simulink model "Problem_8"  (R2020b)
settings: Solver=VariableStepAuto  StartTime=0.0  StopTime=inf  RelTol=1e-3
settings Model: PacingRate=0.028000  Creator=vigne  LastModifiedBy=Yeshwanth

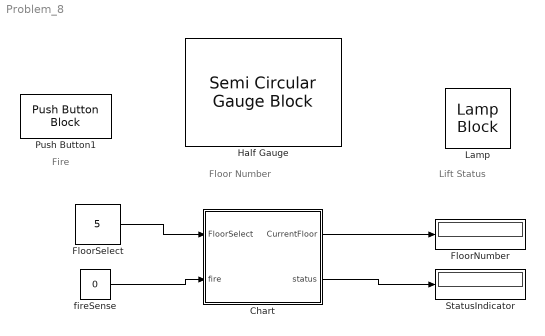
== system Problem_8 ==
  note: Floor Number
  note: Lift Status
  note: Fire
  Chart : Stateflow chart  TreatAsAtomicUnit=on
  FloorNumber : Display
  FloorSelect : Constant  Value=5
  Half Gauge : SemiCircularGaugeBlock  ScaleMax=5  TickInterval=1
  Lamp : LampBlock
  Push Button1 : PushButtonBlock  ButtonText=Fire
  StatusIndicator : Display
  fireSense : Constant  Value=0
  wires:
  FloorSelect/1 -> Chart/1(FloorSelect)
  fireSense/1 -> Chart/2(fire)
  Chart/1(CurrentFloor) -> FloorNumber/1
  Chart/2(status) -> StatusIndicator/1

== stateflow chart Problem_8/Chart ==
  state LiftOperation [parallel]
    entry:
    status=0;
    settings: executionOrder=2
    state LiftFunctionOn
      (history)
      state GroundFloor
        entry:
        status=1;
        during:
        CurrentFloor=0;
        FloorCheck(CurrentFloor);
        exit:
        status=0;
      state FirstFloor
        entry:
        status=1;
        during:
        CurrentFloor=1;
        FloorCheck(CurrentFloor);
        exit:
        status=0;
      state SecondFloor
        entry:
        status=1;
        during:
        CurrentFloor=2;
        FloorCheck(CurrentFloor);
        exit:
        status=0;
        after(1,sec);
      state ThirdFloor
        entry:
        status=1;
        during:
        CurrentFloor=3;
        FloorCheck(CurrentFloor);
        exit:
        status=0;
        after(1,sec);
      state FourthFloor
        entry:
        status=1
        during:
        CurrentFloor=4;
        FloorCheck(CurrentFloor);
        exit:
        status=0;
      state FifthFloor
        entry:
        status=1;
        during:
        CurrentFloor=5;
        FloorCheck(CurrentFloor);
        exit:
        status=0;
      (default) -> GroundFloor
      GroundFloor -> FirstFloor : up
      FirstFloor -> GroundFloor [order 2] : down
      FirstFloor -> SecondFloor [order 1] : up
      SecondFloor -> FirstFloor [order 2] : down
      SecondFloor -> ThirdFloor [order 1] : up
      ThirdFloor -> SecondFloor [order 2] : down
      ThirdFloor -> FourthFloor [order 1] : up
      FourthFloor -> ThirdFloor [order 1] : down
      FourthFloor -> FifthFloor [order 2] : up
      FifthFloor -> FourthFloor : down
    state LiftFunctionOff
      en:
      status=0;
    (default) -> LiftFunctionOn
    LiftFunctionOff -> LiftFunctionOn : [signal==0]
    LiftFunctionOn -> LiftFunctionOff : [signal==1]
  state Alarm [parallel]
    during:
    AlarmStatus = fire;
    FireStatusCheck(AlarmStatus);
    settings: executionOrder=1
  state FireStatusCheck(AlarmSt) [function]
    (default) -> (junction 147)
    (junction 147) -> (junction 148) [order 1] : [AlarmSt ==0]
    (junction 147) -> (junction 149) [order 2] : {signal=1;}
    (junction 148) -> (junction 150) : {signal=0;}
    (junction 150) -> (junction 149)
    (junction 149) -> (junction 151)
  state FloorCheck(Floor) [function]
    (default) -> (junction 62)
    (junction 62) -> (junction 71) [order 3] : [FloorSelect<Floor]{
        | send(down);
        | disp('LiftMovingDown');}
    (junction 62) -> (junction 65) [order 1] : [FloorSelect>Floor]{
        | send(up);
        | disp('LiftMovingUp');}
    (junction 71) -> (junction 86)
    (junction 62) -> (junction 67) [order 2] : [FloorSelect==Floor]{
        | disp('CurrentFloor');}
    (junction 65) -> (junction 89)
    (junction 86) -> (junction 67)
    (junction 89) -> (junction 67)
    (junction 67) -> (junction 69)
  data: AlarmSt function_input; Floor function_input; FloorSelect input; CurrentFloor output; status output; fire input; signal local; AlarmStatus local
  events: up local FUNCTION_CALL_EVENT; down local FUNCTION_CALL_EVENT
